simulink model "IEEE9_16b_fourier_full_cycle"  (R2020a)
settings: Solver=FixedStepAuto  StartTime=0.0  StopTime=5  FixedStep=1/1200/30  MaxStep=1e-4  RelTol=1e-3
libraries: powerlib x33, sps_avr x3, simulink_extras x3
(part 2 of 2)

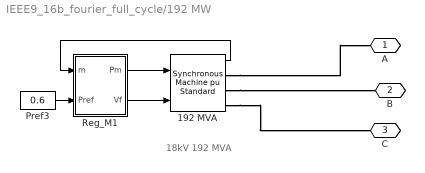
== system IEEE9_16b_fourier_full_cycle/192 MW ==
  note: 18kV 192 MVA
  192 MVA : powerlib/Machines/Synchronous Machine pu Standard  PresetModel=No  MechanicalLoad=Mechanical power Pm  ShowDetailedParameters=on  RotorType=Salient-pole  Units=per unit standard parameters  MeasurementBus=off  NominalParameters="[192e6  18000   60 ]"  Reactances1=[ 31 32 33 34 35 36 37 ]  Reactances2=[ 1.305, 0.296, 0.252, 0.474, 0.243, 0.18 ]  dAxisTimeConstants=Short-circuit  qAxisTimeConstants=Open-circuit  TimeConstants1=[]  TimeConstants2=[]  TimeConstants3=[]  TimeConstants4=[]  TimeConstants5=[ 1.01, 0.053, 0.1 ]  TimeConstants6=[]  TimeConstants7=[]  TimeConstants8=[]  StatorResistance=2.8544e-3  Mechanical="[20 0  32]"  PolePairs=32  InitialConditions=[0 -73.0594 0.600015 0.600015 0.600015 0.71576 -119.284 120.716 1.18255]  SetSaturation=off  Saturation=[0.6404,0.7127,0.8441,0.9214,0.9956,1.082,1.19,1.316,1.457;0.7,0.7698,0.8872,0.9466,0.9969,1.046,1.1,1.151,1.201]  LoadFlowParameters=[1 500000000 0 0 0]  TsPowergui=0  TsBlock=-1  IterativeModel=Trapezoidal non iterative  IterativeDiscreteModel=Trapezoidal non iterative  BusType=PV  Pref=0.6*192e6  Qref=0  Qmin=-Inf  Qmax=Inf  PLF=0  QLF=0
      settings: AttributesFormatString=\n\n
  Pref3 : Constant  Value=0.6
  Reg_M1 : Subsystem
  A : PMIOPort  Side=Right
  B : PMIOPort  Port=2  Side=Right
  C : PMIOPort  Port=3  Side=Right
  wires:
  Reg_M1/1(Pm) -> 192 MVA/1
  192 MVA/1 -> Reg_M1/1(m)
  Reg_M1/2(Vf) -> 192 MVA/2
  Pref3/1 -> Reg_M1/2(Pref)
  connections:
  192 MVA/RConn1 -- A/RConn1
  192 MVA/RConn3 -- C/RConn1
  192 MVA/RConn2 -- B/RConn1

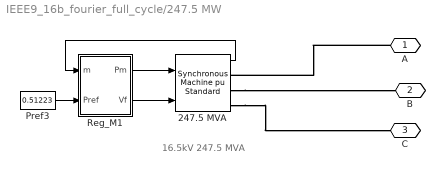
== system IEEE9_16b_fourier_full_cycle/247.5 MW ==
  note: 16.5kV 247.5 MVA
  247.5 MVA : powerlib/Machines/Synchronous Machine pu Standard  PresetModel=No  MechanicalLoad=Mechanical power Pm  ShowDetailedParameters=on  RotorType=Salient-pole  Units=per unit standard parameters  MeasurementBus=off  NominalParameters="[247.5e6  16500   60 ]"  Reactances1=[ 31 32 33 34 35 36 37 ]  Reactances2=[ 1.305, 0.296, 0.252, 0.474, 0.243, 0.18 ]  dAxisTimeConstants=Short-circuit  qAxisTimeConstants=Open-circuit  TimeConstants1=[]  TimeConstants2=[]  TimeConstants3=[]  TimeConstants4=[]  TimeConstants5=[ 1.01, 0.053, 0.1 ]  TimeConstants6=[]  TimeConstants7=[]  TimeConstants8=[]  StatorResistance=2.8544e-3  Mechanical=[20 0 32]  PolePairs=32  InitialConditions=[0 -76.6925 0.514814 0.514814 0.514814 -5.74321 -125.743 114.257 1.19383]  SetSaturation=off  Saturation=[0.6404,0.7127,0.8441,0.9214,0.9956,1.082,1.19,1.316,1.457;0.7,0.7698,0.8872,0.9466,0.9969,1.046,1.1,1.151,1.201]  LoadFlowParameters=[1 500000000 0 0 0]  TsPowergui=0  TsBlock=-1  IterativeModel=Trapezoidal non iterative  IterativeDiscreteModel=Trapezoidal non iterative  BusType=swing  Pref=5e+008  Qref=0  Qmin=-Inf  Qmax=Inf  PLF=0  QLF=0
      settings: AttributesFormatString=\n\n
  Pref3 : Constant  Value=0.51223
  Reg_M1 : Subsystem
  A : PMIOPort  Side=Right
  B : PMIOPort  Port=2  Side=Right
  C : PMIOPort  Port=3  Side=Right
  wires:
  Reg_M1/1(Pm) -> 247.5 MVA/1
  Reg_M1/2(Vf) -> 247.5 MVA/2
  Pref3/1 -> Reg_M1/2(Pref)
  247.5 MVA/1 -> Reg_M1/1(m)
  connections:
  A/RConn1 -- 247.5 MVA/RConn1
  247.5 MVA/RConn2 -- B/RConn1
  247.5 MVA/RConn3 -- C/RConn1

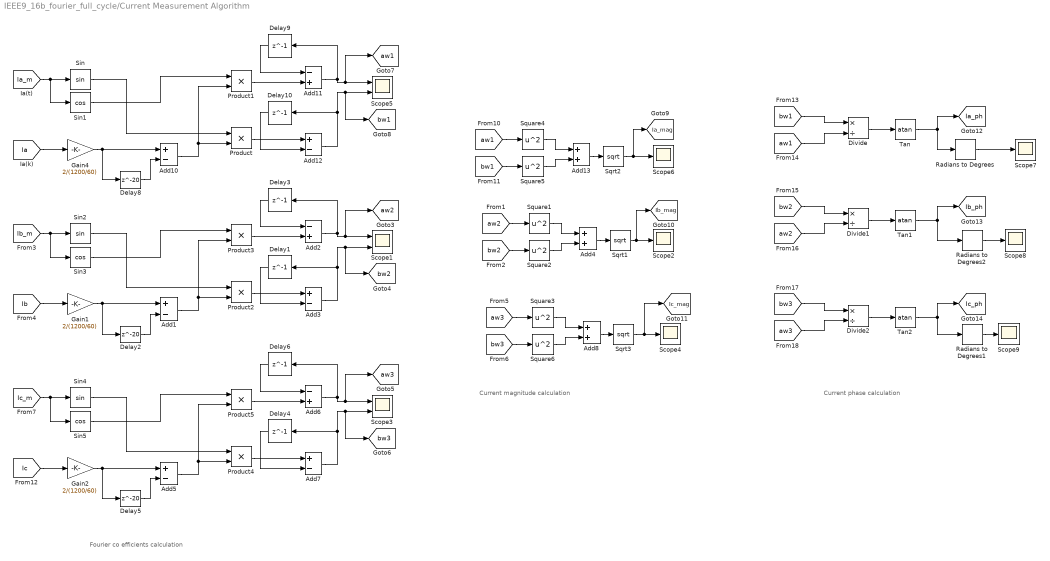
== system IEEE9_16b_fourier_full_cycle/Current Measurement Algorithm ==
  note: Fourier co efficients calculation
  note: Current magnitude calculation
  note: Current phase calculation
  Add{1,3,5,7,10,12} (6 alike) : Sum  Inputs=+-
  Add11 : Sum  Inputs=-+
  Add13 : Sum
  Add2 : Sum  Inputs=-+
  Add4 : Sum
  Add6 : Sum  Inputs=-+
  Add8 : Sum
  Delay{1,3..4,6,9..10} (6 alike) : Delay  DelayLength=1  SampleTime=1/1200
  Delay2 : Delay  DelayLength=20  SampleTime=1/1200
  Delay5 : Delay  DelayLength=20  SampleTime=1/1200
  Delay8 : Delay  DelayLength=20  SampleTime=1/1200
  Divide : Product  Inputs=*/
  Divide1 : Product  Inputs=*/
  Divide2 : Product  Inputs=*/
  Gain1 : Gain  Gain=2/(1200/60)
  Gain2 : Gain  Gain=2/(1200/60)
  Gain4 : Gain  Gain=2/(1200/60)
  Product{,1..5} (6 alike) : Product
  Radians to Degrees : simulink_extras/Transformations/Radians to Degrees
  Radians to Degrees1 : simulink_extras/Transformations/Radians to Degrees
  Radians to Degrees2 : simulink_extras/Transformations/Radians to Degrees
  Scope1 : Scope  NumInputPorts=2
  Scope{2,4,6..9} (6 alike) : Scope
  Scope3 : Scope  NumInputPorts=2
  Scope5 : Scope  NumInputPorts=2
  Sin : Trigonometry
  Sin1 : Trigonometry  Operator=cos
  Sin2 : Trigonometry
  Sin3 : Trigonometry  Operator=cos
  Sin4 : Trigonometry
  Sin5 : Trigonometry  Operator=cos
  Sqrt1 : Sqrt  SaturateOnIntegerOverflow=on
  Sqrt2 : Sqrt  SaturateOnIntegerOverflow=on
  Sqrt3 : Sqrt  SaturateOnIntegerOverflow=on
  Square{1..6} (6 alike) : Math  Operator=square  SaturateOnIntegerOverflow=on
  Tan : Trigonometry  Operator=atan
  Tan1 : Trigonometry  Operator=atan
  Tan2 : Trigonometry  Operator=atan
  tag scope: Ia_mag=global, Ia_ph=global, Ib_mag=global, Ib_ph=global, Ic_mag=global, Ic_ph=global, aw1=global, aw2=global, aw3=global, bw1=global, bw2=global, bw3=global
  wires:
  Gain1/1 -> Add1/1, Delay2/1
  Add5/1 -> Product5/2, Product4/2
  Tan2/1 -> [Ic_ph], Radians to Degrees1/1
  Sqrt2/1 -> [Ia_mag], Scope6/1
  Sin/1 -> Product/1
  Add12/1 -> [bw1], Scope5/2, Delay10/1
  Gain4/1 -> Delay8/1, Add10/1
  Product1/1 -> Add11/2
  Add3/1 -> Delay1/1, Scope1/2, [bw2]
  Add10/1 -> Product1/2, Product/2
  Sqrt1/1 -> [Ib_mag], Scope2/1
  [Ib] -> Gain1/1
  Delay9/1 -> Add11/1
  Delay4/1 -> Add7/2
  [Ia] -> Gain4/1
  Add6/1 -> Delay6/1, [aw3], Scope3/1
  Product/1 -> Add12/1
  [Ib_m] -> Sin2/1, Sin3/1
  Square3/1 -> Add8/1
  Add11/1 -> Delay9/1, [aw1], Scope5/1
  Square6/1 -> Add8/2
  Sqrt3/1 -> [Ic_mag], Scope4/1
  [Ia_m] -> Sin1/1, Sin/1
  Delay10/1 -> Add12/2
  Delay3/1 -> Add2/1
  [Ic_m] -> Sin5/1, Sin4/1
  [bw1] -> Divide/1
  Product3/1 -> Add2/2
  [aw2] -> Divide1/2
  Tan1/1 -> [Ib_ph], Radians to Degrees2/1
  Add2/1 -> Scope1/1, [aw2], Delay3/1
  [aw1] -> Divide/2
  [Ic] -> Gain2/1
  Add1/1 -> Product2/2, Product3/2
  [bw2] -> Divide1/1
  [bw3] -> Square6/1
  Sin4/1 -> Product4/1
  Add4/1 -> Sqrt1/1
  Divide1/1 -> Tan1/1
  Sin3/1 -> Product3/1
  Delay1/1 -> Add3/2
  Square2/1 -> Add4/2
  [bw2] -> Square2/1
  Square1/1 -> Add4/1
  Square4/1 -> Add13/1
  [aw2] -> Square1/1
  [aw3] -> Square3/1
  Divide/1 -> Tan/1
  Product2/1 -> Add3/1
  Delay2/1 -> Add1/2
  Product4/1 -> Add7/1
  Sin2/1 -> Product2/1
  Add8/1 -> Sqrt3/1
  Tan/1 -> [Ia_ph], Radians to Degrees/1
  Add13/1 -> Sqrt2/1
  Square5/1 -> Add13/2
  [aw1] -> Square4/1
  [bw1] -> Square5/1
  Delay5/1 -> Add5/2
  Sin1/1 -> Product1/1
  Gain2/1 -> Delay5/1, Add5/1
  Product5/1 -> Add6/2
  Sin5/1 -> Product5/1
  Add7/1 -> [bw3], Scope3/2, Delay4/1
  Delay6/1 -> Add6/1
  Delay8/1 -> Add10/2
  [bw3] -> Divide2/1
  [aw3] -> Divide2/2
  Divide2/1 -> Tan2/1
  Radians to Degrees/1 -> Scope7/1
  Radians to Degrees1/1 -> Scope9/1
  Radians to Degrees2/1 -> Scope8/1

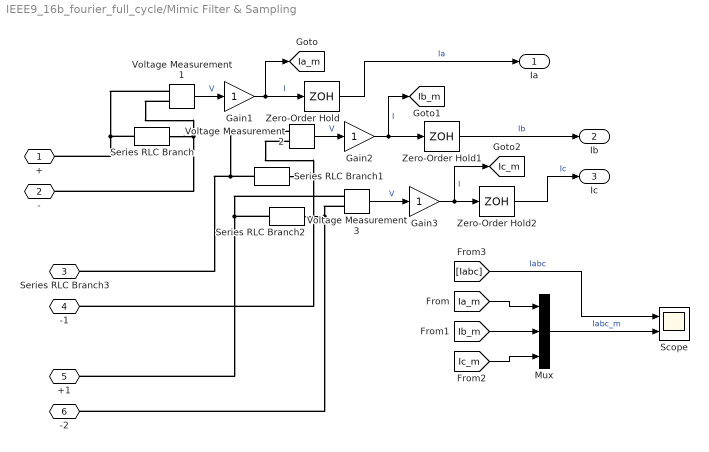
== system IEEE9_16b_fourier_full_cycle/Mimic Filter & Sampling  ==
  Gain1 : Gain
  Gain2 : Gain
  Gain3 : Gain
  Mux : Mux  Inputs=3
  Scope : Scope  NumInputPorts=2
  Series RLC Branch : powerlib/Elements/Series RLC Branch  LConnTagsString=__new0  RConnTagsString=__new0  BranchType=RL  Resistance=0.11727  Inductance=2.634e-3  SetiL0=off  InitialCurrent=0  Capacitance=1e-6  Setx0=off  InitialVoltage=0  Measurements=None
  Series RLC Branch1 : powerlib/Elements/Series RLC Branch  LConnTagsString=__new0  RConnTagsString=__new0  BranchType=RL  Resistance=0.11727  Inductance=2.634e-3  SetiL0=off  InitialCurrent=0  Capacitance=1e-6  Setx0=off  InitialVoltage=0  Measurements=None
  Series RLC Branch2 : powerlib/Elements/Series RLC Branch  LConnTagsString=__new0  RConnTagsString=__new0  BranchType=RL  Resistance=0.11727  Inductance=2.634e-3  SetiL0=off  InitialCurrent=0  Capacitance=1e-6  Setx0=off  InitialVoltage=0  Measurements=None
  Voltage Measurement1 : powerlib/Measurements/Voltage Measurement  PhasorSimulation=off  OutputType=Complex  PSBequivalent=0
  Voltage Measurement2 : powerlib/Measurements/Voltage Measurement  PhasorSimulation=off  OutputType=Complex  PSBequivalent=0
  Voltage Measurement3 : powerlib/Measurements/Voltage Measurement  PhasorSimulation=off  OutputType=Complex  PSBequivalent=0
  Zero-Order Hold : ZeroOrderHold  SampleTime=1/1200
  Zero-Order Hold1 : ZeroOrderHold  SampleTime=1/1200
  Zero-Order Hold2 : ZeroOrderHold  SampleTime=1/1200
  + : PMIOPort  Side=Left
  - : PMIOPort  Port=2  Side=Left
  Series RLC Branch3 : PMIOPort  Port=3  Side=Left
  -1 : PMIOPort  Port=4  Side=Left
  +1 : PMIOPort  Port=5  Side=Left
  -2 : PMIOPort  Port=6  Side=Left
  Ia : Outport
  Ib : Outport  Port=2
  Ic : Outport  Port=3
  tag scope: Ia_m=global, Ib_m=global, Ic_m=global
  wires:
  Voltage Measurement1/1 -> Gain1/1  "V"
  Gain1/1 -> [Ia_m], Zero-Order Hold/1  "I"
  Voltage Measurement2/1 -> Gain2/1  "V"
  Gain2/1 -> [Ib_m], Zero-Order Hold1/1  "I"
  Zero-Order Hold1/1 -> Ib/1  "Ib"
  Voltage Measurement3/1 -> Gain3/1  "V"
  Gain3/1 -> [Ic_m], Zero-Order Hold2/1  "I"
  Zero-Order Hold/1 -> Ia/1  "Ia"
  Zero-Order Hold2/1 -> Ic/1  "Ic"
  [Ib_m] -> Mux/2
  [Ic_m] -> Mux/3
  [Ia_m] -> Mux/1
  Mux/1 -> Scope/2  "Iabc_m"
  [Iabc] -> Scope/1  "Iabc"
  connections:
  Series RLC Branch2/LConn1 -- +1/RConn1 -- Voltage Measurement3/LConn1
  Series RLC Branch/LConn1 -- +/RConn1 -- Voltage Measurement1/LConn1
  Series RLC Branch2/RConn1 -- -2/RConn1 -- Voltage Measurement3/LConn2
  Series RLC Branch1/RConn1 -- -1/RConn1 -- Voltage Measurement2/LConn2
  Voltage Measurement2/LConn1 -- Series RLC Branch3/RConn1 -- Series RLC Branch1/LConn1
  Series RLC Branch/RConn1 -- -/RConn1 -- Voltage Measurement1/LConn2

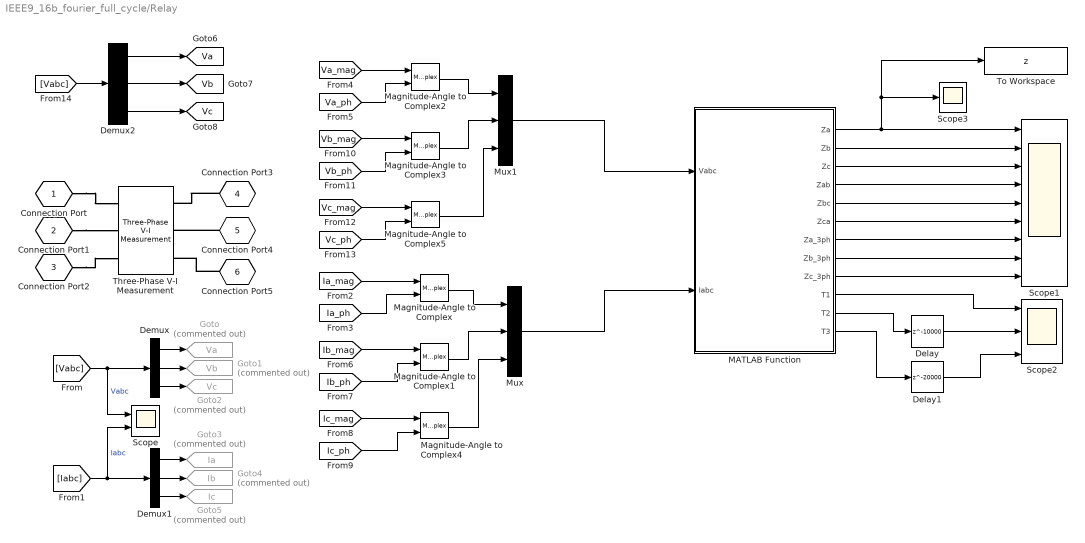
== system IEEE9_16b_fourier_full_cycle/Relay ==
  Delay : Delay  DelayLength=10000  SampleTime=1/1200
  Delay1 : Delay  DelayLength=20000  SampleTime=1/1200
  Demux : Demux  Outputs=3
  Demux1 : Demux  Outputs=3
  Demux2 : Demux  Outputs=3
  Goto : Goto  Commented=on  GotoTag=Va  TagVisibility=global
  Goto1 : Goto  Commented=on  GotoTag=Vb  TagVisibility=global
  Goto2 : Goto  Commented=on  GotoTag=Vc  TagVisibility=global
  Goto3 : Goto  Commented=on  GotoTag=Ia  TagVisibility=global
  Goto4 : Goto  Commented=on  GotoTag=Ib  TagVisibility=global
  Goto5 : Goto  Commented=on  GotoTag=Ic  TagVisibility=global
  MATLAB Function : MATLAB Function  TreatAsAtomicUnit=on
  Magnitude-Angle to Complex{,1..5} (6 alike) : MagnitudeAngleToComplex
  Mux : Mux  Inputs=3
  Mux1 : Mux  Inputs=3
  Scope : Scope  NumInputPorts=2
  Scope1 : Scope  NumInputPorts=9
  Scope2 : Scope  NumInputPorts=3
  Scope3 : Scope
  Three-Phase V-I Measurement : powerlib/Measurements/Three-Phase V-I Measurement  VoltageMeasurement=phase-to-ground  SetLabelV=on  LabelV=Vabc  Vpu=off  VpuLL=off  CurrentMeasurement=yes  SetLabelI=on  LabelI=Iabc  Ipu=off  Pbase=100e6  Vbase=500e3  OutputType=Complex  PhasorSimulation=off  PSBequivalent=0
  To Workspace : ToWorkspace  VariableName=z  SampleTime=-1
  Connection Port : PMIOPort  Tag=PMCPort  Side=Left
  Connection Port1 : PMIOPort  Tag=PMCPort  Port=2  Side=Left
  Connection Port2 : PMIOPort  Tag=PMCPort  Port=3  Side=Left
  Connection Port3 : PMIOPort  Tag=PMCPort  Port=4  Side=Right
  Connection Port4 : PMIOPort  Tag=PMCPort  Port=5  Side=Right
  Connection Port5 : PMIOPort  Tag=PMCPort  Port=6  Side=Right
  tag scope: Va=global, Vb=global, Vc=global
  wires:
  Demux1/3 -> Goto5/1
  Demux1/1 -> Goto3/1
  Demux/3 -> Goto2/1
  Demux/1 -> Goto/1
  Demux/2 -> Goto1/1
  [Iabc] -> Scope/2, Demux1/1  "Iabc"
  [Vabc] -> Scope/1, Demux/1  "Vabc"
  Demux1/2 -> Goto4/1
  MATLAB Function/1(Za) -> To Workspace/1, Scope3/1, Scope1/1
  MATLAB Function/2(Zb) -> Scope1/2
  MATLAB Function/3(Zc) -> Scope1/3
  MATLAB Function/4(Zab) -> Scope1/4
  MATLAB Function/5(Zbc) -> Scope1/5
  MATLAB Function/6(Zca) -> Scope1/6
  MATLAB Function/10(T1) -> Scope2/1
  Mux/1 -> MATLAB Function/2(Iabc)
  MATLAB Function/11(T2) -> Delay/1
  MATLAB Function/12(T3) -> Delay1/1
  Delay/1 -> Scope2/2
  Delay1/1 -> Scope2/3
  MATLAB Function/7(Za_3ph) -> Scope1/7
  MATLAB Function/8(Zb_3ph) -> Scope1/8
  MATLAB Function/9(Zc_3ph) -> Scope1/9
  [Ia_mag] -> Magnitude-Angle to Complex/1
  [Ia_ph] -> Magnitude-Angle to Complex/2
  [Ib_ph] -> Magnitude-Angle to Complex1/2
  [Ib_mag] -> Magnitude-Angle to Complex1/1
  [Ic_mag] -> Magnitude-Angle to Complex4/1
  [Ic_ph] -> Magnitude-Angle to Complex4/2
  Magnitude-Angle to Complex/1 -> Mux/1
  Magnitude-Angle to Complex1/1 -> Mux/2
  Magnitude-Angle to Complex4/1 -> Mux/3
  Magnitude-Angle to Complex5/1 -> Mux1/3
  Magnitude-Angle to Complex3/1 -> Mux1/2
  Magnitude-Angle to Complex2/1 -> Mux1/1
  [Vc_ph] -> Magnitude-Angle to Complex5/2
  [Vc_mag] -> Magnitude-Angle to Complex5/1
  [Vb_mag] -> Magnitude-Angle to Complex3/1
  [Vb_ph] -> Magnitude-Angle to Complex3/2
  [Va_ph] -> Magnitude-Angle to Complex2/2
  [Va_mag] -> Magnitude-Angle to Complex2/1
  Mux1/1 -> MATLAB Function/1(Vabc)
  [Vabc] -> Demux2/1
  Demux2/1 -> [Va]
  Demux2/2 -> [Vb]
  Demux2/3 -> [Vc]
  connections:
  Connection Port/RConn1 -- Three-Phase V-I Measurement/LConn1
  Connection Port1/RConn1 -- Three-Phase V-I Measurement/LConn2
  Connection Port2/RConn1 -- Three-Phase V-I Measurement/LConn3
  Connection Port3/RConn1 -- Three-Phase V-I Measurement/RConn1
  Connection Port4/RConn1 -- Three-Phase V-I Measurement/RConn2
  Connection Port5/RConn1 -- Three-Phase V-I Measurement/RConn3

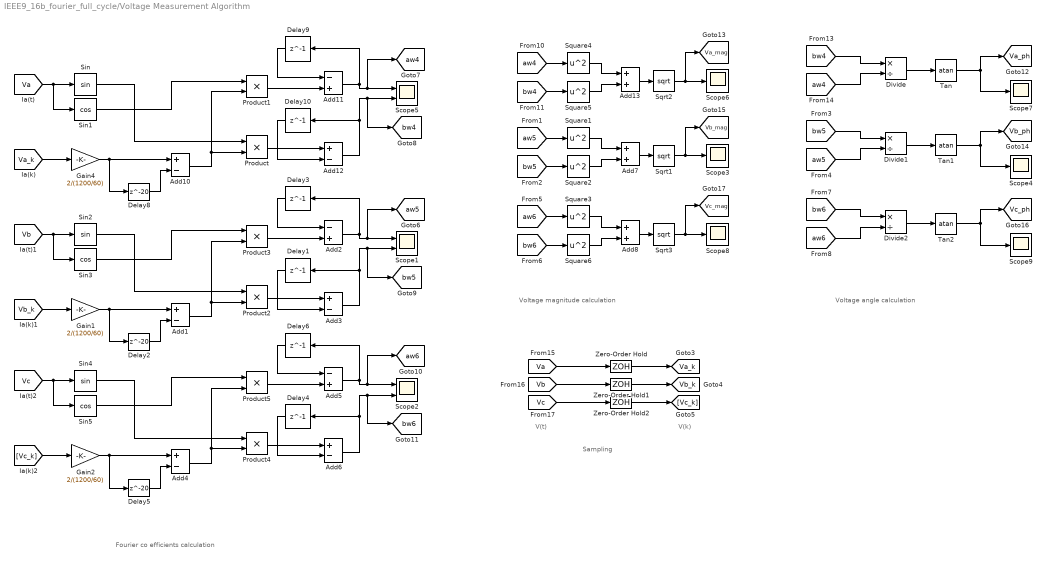
== system IEEE9_16b_fourier_full_cycle/Voltage Measurement Algorithm ==
  note: V(t)
  note: V(k)
  note: Voltage magnitude calculation
  note: Fourier co efficients calculation
  note: Voltage angle calculation
  note: Sampling
  Add{1,3..4,6,10,12} (6 alike) : Sum  Inputs=+-
  Add11 : Sum  Inputs=-+
  Add13 : Sum
  Add2 : Sum  Inputs=-+
  Add5 : Sum  Inputs=-+
  Add7 : Sum
  Add8 : Sum
  Delay{1,3..4,6,9..10} (6 alike) : Delay  DelayLength=1  SampleTime=1/1200
  Delay2 : Delay  DelayLength=20  SampleTime=1/1200
  Delay5 : Delay  DelayLength=20  SampleTime=1/1200
  Delay8 : Delay  DelayLength=20  SampleTime=1/1200
  Divide : Product  Inputs=*/
  Divide1 : Product  Inputs=*/
  Divide2 : Product  Inputs=*/
  Gain1 : Gain  Gain=2/(1200/60)
  Gain2 : Gain  Gain=2/(1200/60)
  Gain4 : Gain  Gain=2/(1200/60)
  Product{,1..5} (6 alike) : Product
  Scope1 : Scope  NumInputPorts=2
  Scope2 : Scope  NumInputPorts=2
  Scope{3..4,6..9} (6 alike) : Scope
  Scope5 : Scope  NumInputPorts=2
  Sin : Trigonometry
  Sin1 : Trigonometry  Operator=cos
  Sin2 : Trigonometry
  Sin3 : Trigonometry  Operator=cos
  Sin4 : Trigonometry
  Sin5 : Trigonometry  Operator=cos
  Sqrt1 : Sqrt  SaturateOnIntegerOverflow=on
  Sqrt2 : Sqrt  SaturateOnIntegerOverflow=on
  Sqrt3 : Sqrt  SaturateOnIntegerOverflow=on
  Square{1..6} (6 alike) : Math  Operator=square  SaturateOnIntegerOverflow=on
  Tan : Trigonometry  Operator=atan
  Tan1 : Trigonometry  Operator=atan
  Tan2 : Trigonometry  Operator=atan
  Zero-Order Hold : ZeroOrderHold  SampleTime=1/1200
  Zero-Order Hold1 : ZeroOrderHold  SampleTime=1/1200
  Zero-Order Hold2 : ZeroOrderHold  SampleTime=1/1200
  tag scope: Va_k=global, Va_mag=global, Va_ph=global, Vb_k=global, Vb_mag=global, Vb_ph=global, Vc_mag=global, Vc_ph=global, aw4=global, aw5=global, aw6=global, bw4=global, bw5=global, bw6=global
  wires:
  Sin2/1 -> Product2/1
  Tan/1 -> [Va_ph], Scope7/1
  Square5/1 -> Add13/2
  Gain2/1 -> Delay5/1, Add4/1
  [Vc] -> Sin5/1, Sin4/1
  Add6/1 -> [bw6], Scope2/2, Delay4/1
  Add13/1 -> Sqrt2/1
  Add8/1 -> Sqrt3/1
  Divide/1 -> Tan/1
  Product4/1 -> Add6/1
  Sin/1 -> Product/1
  Sin1/1 -> Product1/1
  Delay1/1 -> Add3/2
  [bw6] -> Divide2/1
  Tan2/1 -> [Vc_ph], Scope9/1
  [Va] -> Sin1/1, Sin/1
  Product1/1 -> Add11/2
  Square4/1 -> Add13/1
  [aw6] -> Divide2/2
  [Vc_k] -> Gain2/1
  [aw4] -> Square4/1
  Sqrt2/1 -> [Va_mag], Scope6/1
  [Vb_k] -> Gain1/1
  Zero-Order Hold1/1 -> [Vb_k]
  [aw4] -> Divide/2
  [aw6] -> Square3/1
  Add4/1 -> Product5/2, Product4/2
  Add3/1 -> Delay1/1, Scope1/2, [bw5]
  [bw4] -> Square5/1
  Sin4/1 -> Product4/1
  Product3/1 -> Add2/2
  [Vb] -> Sin2/1, Sin3/1
  [bw4] -> Divide/1
  Delay5/1 -> Add4/2
  Zero-Order Hold2/1 -> [Vc_k]
  [Vb] -> Zero-Order Hold1/1
  Delay3/1 -> Add2/1
  [Va_k] -> Gain4/1
  Add2/1 -> Scope1/1, [aw5], Delay3/1
  Gain1/1 -> Add1/1, Delay2/1
  Add1/1 -> Product2/2, Product3/2
  Add5/1 -> Delay6/1, [aw6], Scope2/1
  Product2/1 -> Add3/1
  Sin3/1 -> Product3/1
  [Vc] -> Zero-Order Hold2/1
  Sqrt1/1 -> Scope3/1, [Vb_mag]
  Delay2/1 -> Add1/2
  Zero-Order Hold/1 -> [Va_k]
  Add12/1 -> [bw4], Scope5/2, Delay10/1
  Square3/1 -> Add8/1
  [Va] -> Zero-Order Hold/1
  Delay4/1 -> Add6/2
  Delay6/1 -> Add5/1
  Add10/1 -> Product1/2, Product/2
  Product5/1 -> Add5/2
  Gain4/1 -> Delay8/1, Add10/1
  Delay10/1 -> Add12/2
  Add11/1 -> Delay9/1, [aw4], Scope5/1
  Product/1 -> Add12/1
  Delay9/1 -> Add11/1
  Delay8/1 -> Add10/2
  Sin5/1 -> Product5/1
  Sqrt3/1 -> [Vc_mag], Scope8/1
  Square6/1 -> Add8/2
  Divide2/1 -> Tan2/1
  [bw6] -> Square6/1
  [bw5] -> Divide1/1
  Tan1/1 -> Scope4/1, [Vb_ph]
  Add7/1 -> Sqrt1/1
  Square2/1 -> Add7/2
  [aw5] -> Divide1/2
  Square1/1 -> Add7/1
  [bw5] -> Square2/1
  [aw5] -> Square1/1
  Divide1/1 -> Tan1/1

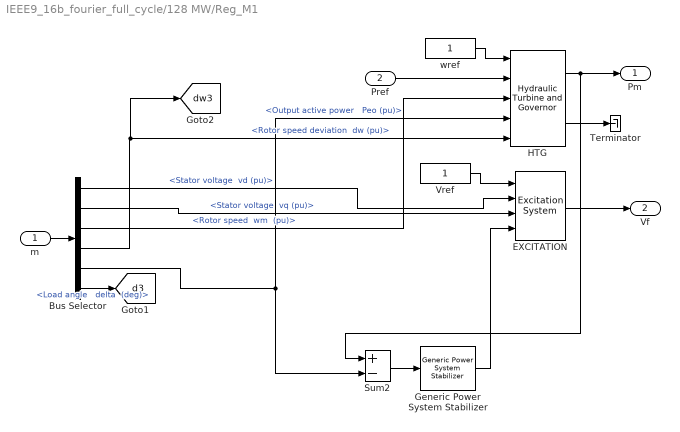
== system IEEE9_16b_fourier_full_cycle/128 MW/Reg_M1 ==
  m : Inport
  Pref : Inport  Port=2
  Bus Selector : BusSelector  OutputSignals="dq0 components.Stator voltage  vd (pu),dq0 components.Stator voltage  vq (pu),Mechanical.Rotor speed  wm  (pu),Mechanical.Rotor speed deviation  dw (pu),Output active power   Peo (pu),Load angle   delta  (deg)"
  EXCITATION : sps_avr/Excitation System  tr=20e-3  reg=[ 200, 0.001 ]  exc=[ 1, 0 ]  tgr=[ 0, 0 ]  damp=[ 0.001, 0.1 ]  sat=[ 0, 0 ]  lim="[ 0,  7, 0 ]"  v0=[1 1.1034]
      settings: SourceProductBaseCode=PS
  Generic Power System Stabilizer : powerlib/Machines/Generic Power System Stabilizer  Tsensor=15e-3  K=2.5  Twashout=1  Tleadlag1="[0.06  1]"  Tleadlag2="[0  0]"  VSlimits=[-0.15 0.15]  Vinit=0  Plot_On=off  MagdB_On=on  FreqRange=logspace(-2,2,500)
      settings: SourceProductBaseCode=PS
  HTG : powerlib/Machines/Hydraulic Turbine and Governor  sm="[ 10/3  0.07 ]"  gate="[  0.01  0.97518  -0.1  0.1 ]"  reg="[  0.05  1.163  0.105  0  0.01  ]"  hyd="[  0  2.67  ]"  dref=0  po=0.60104
      settings: SourceProductBaseCode=PS
  Sum2 : Sum  Inputs=+-  InputSameDT=on  SaturateOnIntegerOverflow=on  OutDataTypeStr=Inherit: Same as first input
  Terminator : Terminator
  Vref : Constant
  wref : Constant
  Pm : Outport  InitialOutput=0
  Vf : Outport  Port=2  InitialOutput=0
  tag scope: d3=global, dw3=global
  wires:
  HTG/2 -> Terminator/1
  Vref/1 -> EXCITATION/1
  m/1 -> Bus Selector/1
  Bus Selector/4 -> [dw3], HTG/5  "<Rotor speed deviation  dw (pu)>"
  Bus Selector/5 -> HTG/4, Sum2/2  "<Output active power   Peo (pu)>"
  Bus Selector/3 -> HTG/3  "<Rotor speed  wm  (pu)>"
  Pref/1 -> HTG/2
  wref/1 -> HTG/1
  HTG/1 -> Pm/1, Sum2/1
  Bus Selector/2 -> EXCITATION/3  "<Stator voltage  vq (pu)>"
  EXCITATION/1 -> Vf/1
  Bus Selector/1 -> EXCITATION/2  "<Stator voltage  vd (pu)>"
  Generic Power System Stabilizer/1 -> EXCITATION/4
  Sum2/1 -> Generic Power System Stabilizer/1
  Bus Selector/6 -> [d3]  "<Load angle   delta  (deg)>"

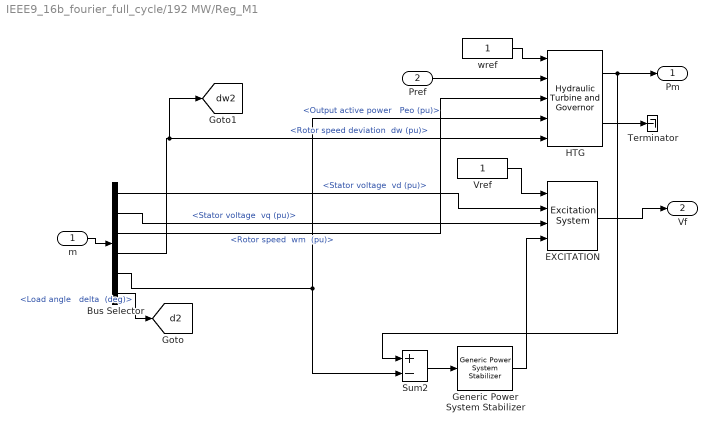
== system IEEE9_16b_fourier_full_cycle/192 MW/Reg_M1 ==
  m : Inport
  Pref : Inport  Port=2
  Bus Selector : BusSelector  OutputSignals="dq0 components.Stator voltage  vd (pu),dq0 components.Stator voltage  vq (pu),Mechanical.Rotor speed  wm  (pu),Mechanical.Rotor speed deviation  dw (pu),Output active power   Peo (pu),Load angle   delta  (deg)"
  EXCITATION : sps_avr/Excitation System  tr=20e-3  reg=[ 200, 0.001 ]  exc=[ 1, 0 ]  tgr=[ 0, 0 ]  damp=[ 0.001, 0.1 ]  sat=[ 0, 0 ]  lim="[ 0,  7, 0 ]"  v0=[1 1.1826]
      settings: SourceProductBaseCode=PS
  Generic Power System Stabilizer : powerlib/Machines/Generic Power System Stabilizer  Tsensor=15e-3  K=2.5  Twashout=1  Tleadlag1="[0.06  1]"  Tleadlag2="[0  0]"  VSlimits=[-0.15 0.15]  Vinit=0  Plot_On=off  MagdB_On=on  FreqRange=logspace(-2,2,500)
      settings: SourceProductBaseCode=PS
  HTG : powerlib/Machines/Hydraulic Turbine and Governor  sm="[ 10/3  0.07 ]"  gate="[  0.01  0.97518  -0.1  0.1 ]"  reg="[  0.05  1.163  0.105  0  0.01  ]"  hyd="[  0  2.67  ]"  dref=0  po=0.60103
      settings: SourceProductBaseCode=PS
  Sum2 : Sum  Inputs=+-  InputSameDT=on  SaturateOnIntegerOverflow=on  OutDataTypeStr=Inherit: Same as first input
  Terminator : Terminator
  Vref : Constant
  wref : Constant
  Pm : Outport  InitialOutput=0
  Vf : Outport  Port=2  InitialOutput=0
  tag scope: d2=global, dw2=global
  wires:
  HTG/2 -> Terminator/1
  Vref/1 -> EXCITATION/1
  m/1 -> Bus Selector/1
  Bus Selector/4 -> [dw2], HTG/5  "<Rotor speed deviation  dw (pu)>"
  Bus Selector/5 -> HTG/4, Sum2/2  "<Output active power   Peo (pu)>"
  Bus Selector/3 -> HTG/3  "<Rotor speed  wm  (pu)>"
  Pref/1 -> HTG/2
  wref/1 -> HTG/1
  HTG/1 -> Pm/1, Sum2/1
  Bus Selector/2 -> EXCITATION/3  "<Stator voltage  vq (pu)>"
  EXCITATION/1 -> Vf/1
  Bus Selector/1 -> EXCITATION/2  "<Stator voltage  vd (pu)>"
  Generic Power System Stabilizer/1 -> EXCITATION/4
  Sum2/1 -> Generic Power System Stabilizer/1
  Bus Selector/6 -> [d2]  "<Load angle   delta  (deg)>"

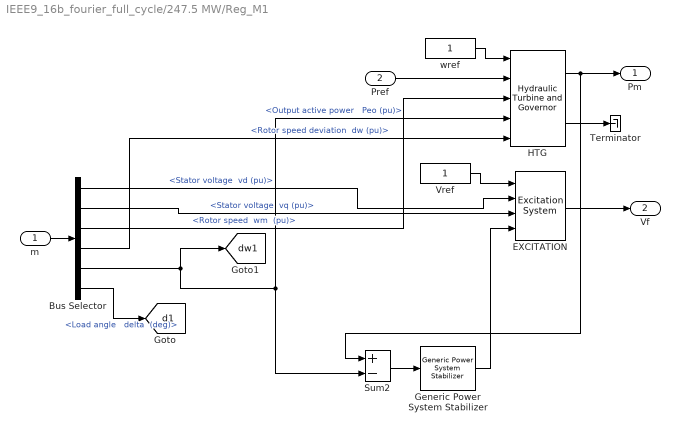
== system IEEE9_16b_fourier_full_cycle/247.5 MW/Reg_M1 ==
  m : Inport
  Pref : Inport  Port=2
  Bus Selector : BusSelector  OutputSignals="dq0 components.Stator voltage  vd (pu),dq0 components.Stator voltage  vq (pu),Mechanical.Rotor speed  wm  (pu),Mechanical.Rotor speed deviation  dw (pu),Output active power   Peo (pu),Load angle   delta  (deg)"
  EXCITATION : sps_avr/Excitation System  tr=20e-3  reg=[ 200, 0.001 ]  exc=[ 1, 0 ]  tgr=[ 0, 0 ]  damp=[ 0.001, 0.1 ]  sat=[ 0, 0 ]  lim="[ 0,  7, 0 ]"  v0=[1 1.1938]
      settings: SourceProductBaseCode=PS
  Generic Power System Stabilizer : powerlib/Machines/Generic Power System Stabilizer  Tsensor=15e-3  K=2.5  Twashout=1  Tleadlag1="[0.06  1]"  Tleadlag2="[0  0]"  VSlimits=[-0.15 0.15]  Vinit=0  Plot_On=off  MagdB_On=on  FreqRange=logspace(-2,2,500)
      settings: SourceProductBaseCode=PS
  HTG : powerlib/Machines/Hydraulic Turbine and Governor  sm="[ 10/3  0.07 ]"  gate="[  0.01  0.97518  -0.1  0.1 ]"  reg="[  0.05  1.163  0.105  0  0.01  ]"  hyd="[  0  2.67  ]"  dref=0  po=0.51299
      settings: SourceProductBaseCode=PS
  Sum2 : Sum  Inputs=+-  InputSameDT=on  SaturateOnIntegerOverflow=on  OutDataTypeStr=Inherit: Same as first input
  Terminator : Terminator
  Vref : Constant
  wref : Constant
  Pm : Outport  InitialOutput=0
  Vf : Outport  Port=2  InitialOutput=0
  tag scope: d1=global, dw1=global
  wires:
  HTG/2 -> Terminator/1
  Vref/1 -> EXCITATION/1
  m/1 -> Bus Selector/1
  Bus Selector/4 -> HTG/5  "<Rotor speed deviation  dw (pu)>"
  Bus Selector/5 -> [dw1], HTG/4, Sum2/2  "<Output active power   Peo (pu)>"
  Bus Selector/3 -> HTG/3  "<Rotor speed  wm  (pu)>"
  Pref/1 -> HTG/2
  wref/1 -> HTG/1
  HTG/1 -> Pm/1, Sum2/1
  Bus Selector/2 -> EXCITATION/3  "<Stator voltage  vq (pu)>"
  EXCITATION/1 -> Vf/1
  Bus Selector/1 -> EXCITATION/2  "<Stator voltage  vd (pu)>"
  Generic Power System Stabilizer/1 -> EXCITATION/4
  Sum2/1 -> Generic Power System Stabilizer/1
  Bus Selector/6 -> [d1]  "<Load angle   delta  (deg)>"

== matlab function IEEE9_16b_fourier_full_cycle/Relay/MATLAB Function ==
  settings: updateMethod=DISCRETE
  data: Vabc input; Za output; Iabc input; Zb output; Zc output; Zab output; Zbc output; Zca output; Za_3ph output; Zb_3ph output; Zc_3ph output; T1 output; T2 output; T3 output
function [Za, Zb, Zc, Zab, Zbc, Zca, Za_3ph, Zb_3ph, Zc_3ph, T1, T2, T3] = fcn(Vabc, Iabc)
 
persistent init C1 C2 C3 r1 r2 r3 trip1 trip2 trip3 k
if isempty(init)  
    trip1 = false; trip2 = false; trip3 = false;
    Zline = 100*(0.0449 + 1i*2*pi*60*1.01e-3);
    Z0_line = 100*(0.11241 + 1i*60*2.02e-3*2*pi);
    k = (Z0_line - Zline)./Zline;
    Z1 = 0.80*Zline;
    Z2 = 1.2*Zline;
    Z3 = 2*abs(Zline)*exp(1i*80*pi/180);
    C1 = Z1/2; C2 = Z2/2; C3 = Z3/2;
    r1 = abs(C1); r2 = abs(C2); r3 = abs(C3);
    MTA1 = angle(Z1);
    MTA2 = angle(Z2);
    MTA3 = 80*pi/180;
    init = 1;
    
%     circle(real(C1),imag(C1),r1)
%     circle(real(C2),imag(C2),r2)
%     circle(real(C3),imag(C3),r3)
end

Va = Vabc(1); Vb = Vabc(2); Vc = Vabc(3);
Ia = Iabc(1); Ib = Iabc(2); Ic =Iabc(3);
Io = (Ia+Ib+Ic)/3;

Za = Va/(Ia+k*Io);
Zb = Vb/(Ib+k*Io);
Zc = Vc/(Ic+k*Io);
Zab = (Va-Vb)/(Ia-Ib);
Zbc = (Vb-Vc)/(Ib-Ic);
Zca = (Vc-Va)/(Ic-Ia);
Za_3ph = Va/Ia;
Zb_3ph = Vb/Ib;
Zc_3ph = Vc/Ic;

if any([abs(Za-C1),abs(Zb-C1),abs(Zc-C1),abs(Zab-C1),abs(Zbc-C1),abs(Zca-C1),abs(Za_3ph-C1),abs(Zb_3ph-C1),abs(Zc_3ph-C1)] <= r1)
    trip1 = true;
elseif any([abs(Za-C2),abs(Zb-C2),abs(Zc-C2),abs(Zab-C2),abs(Zbc-C2),abs(Zca-C2),abs(Za_3ph-C2),abs(Zb_3ph-C2),abs(Zc_3ph-C2)] <= r2)
    trip2 = true;
elseif any([abs(Za-C3),abs(Zb-C3),abs(Zc-C3),abs(Zab-C3),abs(Zbc-C3),abs(Zca-C3),abs(Za_3ph-C3),abs(Zb_3ph-C3),abs(Zc_3ph-C3)] <= r3)
    trip3 = true;
end

T1 =trip1; T2 = trip2; T3 = trip3;
end
